simulink model "Filter_testaus_uusi"  (R2017b)
settings: Solver=FixedStepDiscrete  StartTime=0.0  StopTime=10  FixedStep=1/44100  RelTol=1e-3
(part 1 of 4)
settings Model: Creator=Jouni  LastModifiedBy=Jouni
settings CodeAppCC: StateflowObjectComments=on
settings ConfigComp: PLC_TargetIDE=twincat3  PLC_GenerateReport=off  PLC_LaunchReport=off

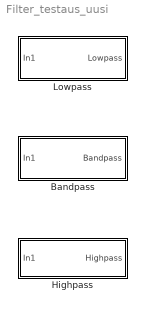
== system Filter_testaus_uusi ==
  Bandpass : Subsystem  TreatAsAtomicUnit=on
  Highpass : Subsystem  TreatAsAtomicUnit=on
  Lowpass : Subsystem  TreatAsAtomicUnit=on

== system Filter_testaus_uusi/Bandpass ==
  In1 : Inport
  BandpassH : Subsystem
  Complex to Real-Imag1 : ComplexToRealImag
  Sum3 : Sum
  Bandpass : Outport
  wires:
  Complex to Real-Imag1/2 -> Sum3/2
  BandpassH/1(Out1) -> Complex to Real-Imag1/1
  Sum3/1 -> Bandpass/1  "Bandpass"
  Complex to Real-Imag1/1 -> Sum3/1
  In1/1 -> BandpassH/1(In1)

== system Filter_testaus_uusi/Highpass ==
  In1 : Inport
  Complex to Real-Imag2 : ComplexToRealImag
  HighpassH : Subsystem
  Sum4 : Sum
  Highpass : Outport
  wires:
  Complex to Real-Imag2/2 -> Sum4/2
  HighpassH/1(Out1) -> Complex to Real-Imag2/1
  Complex to Real-Imag2/1 -> Sum4/1
  Sum4/1 -> Highpass/1  "Highpass"
  In1/1 -> HighpassH/1(In1)

== system Filter_testaus_uusi/Lowpass ==
  In1 : Inport
  Complex to Real-Imag : ComplexToRealImag
  Filter1 : Subsystem  Tag=FilterWizardSubSystem  TreatAsAtomicUnit=on
      settings: ErrorFcn=dspFilterRealizedInBasicElemsAlgLoopErrFcnCallback
  Gain : Gain  Gain=0.75
  LowpassH : Subsystem
  Sum2 : Sum
  Lowpass : Outport
  wires:
  Complex to Real-Imag/2 -> Sum2/2
  LowpassH/1(Out1) -> Complex to Real-Imag/1
  Complex to Real-Imag/1 -> Sum2/1
  Gain/1 -> Filter1/1(Input)
  Sum2/1 -> Lowpass/1  "Lowpass"
  Filter1/1(Output) -> LowpassH/1(In1)
  In1/1 -> Gain/1

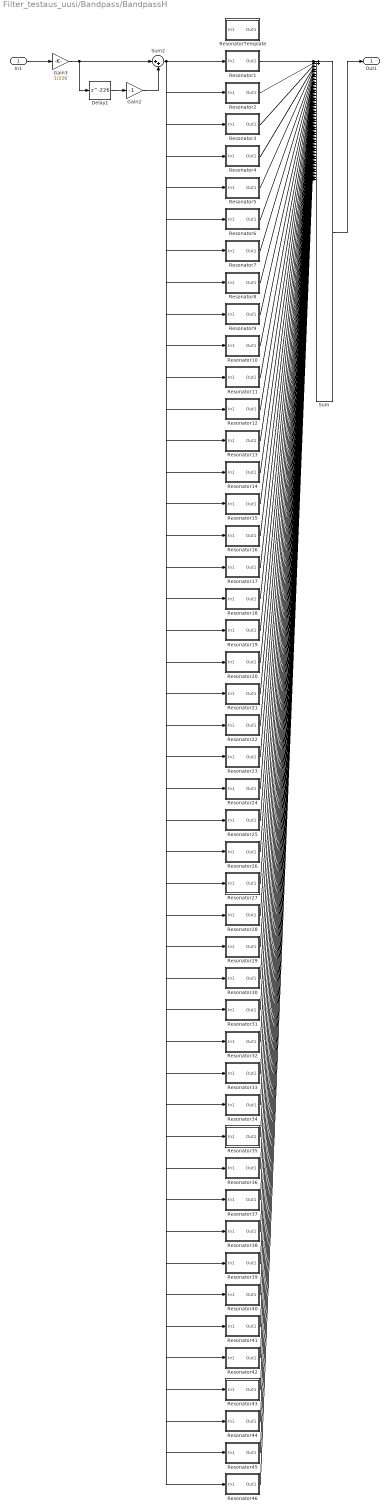
== system Filter_testaus_uusi/Bandpass/BandpassH ==
  In1 : Inport
  Delay1 : Delay  DelayLength=226
  Gain2 : Gain  Gain=-1
  Gain3 : Gain  Gain=1/226
  Resonator1 : Subsystem
  Resonator10 : Subsystem
  Resonator11 : Subsystem
  Resonator12 : Subsystem
  Resonator13 : Subsystem
  Resonator14 : Subsystem
  Resonator15 : Subsystem
  Resonator16 : Subsystem
  Resonator17 : Subsystem
  Resonator18 : Subsystem
  Resonator19 : Subsystem
  Resonator2 : Subsystem
  Resonator20 : Subsystem
  Resonator21 : Subsystem
  Resonator22 : Subsystem
  Resonator23 : Subsystem
  Resonator24 : Subsystem
  Resonator25 : Subsystem
  Resonator26 : Subsystem
  Resonator27 : Subsystem
  Resonator28 : Subsystem
  Resonator29 : Subsystem
  Resonator3 : Subsystem
  Resonator30 : Subsystem
  Resonator31 : Subsystem
  Resonator32 : Subsystem
  Resonator33 : Subsystem
  Resonator34 : Subsystem
  Resonator35 : Subsystem
  Resonator36 : Subsystem
  Resonator37 : Subsystem
  Resonator38 : Subsystem
  Resonator39 : Subsystem
  Resonator4 : Subsystem
  Resonator40 : Subsystem
  Resonator41 : Subsystem
  Resonator42 : Subsystem
  Resonator43 : Subsystem
  Resonator44 : Subsystem
  Resonator45 : Subsystem
  Resonator46 : Subsystem
  Resonator5 : Subsystem
  Resonator6 : Subsystem
  Resonator7 : Subsystem
  Resonator8 : Subsystem
  Resonator9 : Subsystem
  ResonatorTemplate : Subsystem
  Sum : Sum  Inputs=<binary blob, 130 chars, not shown>
  Sum2 : Sum  Inputs=|++
  Out1 : Outport
  wires:
  Delay1/1 -> Gain2/1
  Gain3/1 -> Sum2/1, Delay1/1
  Gain2/1 -> Sum2/2
  In1/1 -> Gain3/1
  Sum/1 -> Out1/1
  Sum2/1 -> Resonator1/1(In1), Resonator2/1(In1), Resonator3/1(In1), Resonator4/1(In1), Resonator5/1(In1), Resonator6/1(In1), Resonator7/1(In1), Resonator8/1(In1), Resonator9/1(In1), Resonator10/1(In1), Resonator11/1(In1), Resonator12/1(In1), Resonator13/1(In1), Resonator14/1(In1), Resonator15/1(In1), Resonator16/1(In1), Resonator17/1(In1), Resonator18/1(In1), Resonator19/1(In1), Resonator20/1(In1), Resonator21/1(In1), Resonator22/1(In1), Resonator23/1(In1), Resonator24/1(In1), Resonator25/1(In1), Resonator26/1(In1), Resonator27/1(In1), Resonator28/1(In1), Resonator29/1(In1), Resonator30/1(In1), Resonator31/1(In1), Resonator32/1(In1), Resonator33/1(In1), Resonator34/1(In1), Resonator35/1(In1), Resonator36/1(In1), Resonator37/1(In1), Resonator38/1(In1), Resonator39/1(In1), Resonator40/1(In1), Resonator41/1(In1), Resonator42/1(In1), Resonator43/1(In1), Resonator44/1(In1), Resonator45/1(In1), Resonator46/1(In1)
  Resonator1/1(Out1) -> Sum/1
  Resonator2/1(Out1) -> Sum/2
  Resonator3/1(Out1) -> Sum/3
  Resonator4/1(Out1) -> Sum/4
  Resonator5/1(Out1) -> Sum/5
  Resonator6/1(Out1) -> Sum/6
  Resonator7/1(Out1) -> Sum/7
  Resonator8/1(Out1) -> Sum/8
  Resonator9/1(Out1) -> Sum/9
  Resonator10/1(Out1) -> Sum/10
  Resonator11/1(Out1) -> Sum/11
  Resonator12/1(Out1) -> Sum/12
  Resonator13/1(Out1) -> Sum/13
  Resonator14/1(Out1) -> Sum/14
  Resonator15/1(Out1) -> Sum/15
  Resonator16/1(Out1) -> Sum/16
  Resonator17/1(Out1) -> Sum/17
  Resonator18/1(Out1) -> Sum/18
  Resonator19/1(Out1) -> Sum/19
  Resonator20/1(Out1) -> Sum/20
  Resonator21/1(Out1) -> Sum/21
  Resonator22/1(Out1) -> Sum/22
  Resonator23/1(Out1) -> Sum/23
  Resonator24/1(Out1) -> Sum/24
  Resonator25/1(Out1) -> Sum/25
  Resonator26/1(Out1) -> Sum/26
  Resonator27/1(Out1) -> Sum/27
  Resonator28/1(Out1) -> Sum/28
  Resonator29/1(Out1) -> Sum/29
  Resonator30/1(Out1) -> Sum/30
  Resonator31/1(Out1) -> Sum/31
  Resonator32/1(Out1) -> Sum/32
  Resonator33/1(Out1) -> Sum/33
  Resonator34/1(Out1) -> Sum/34
  Resonator35/1(Out1) -> Sum/35
  Resonator36/1(Out1) -> Sum/36
  Resonator37/1(Out1) -> Sum/37
  Resonator38/1(Out1) -> Sum/38
  Resonator39/1(Out1) -> Sum/39
  Resonator40/1(Out1) -> Sum/40
  Resonator41/1(Out1) -> Sum/41
  Resonator42/1(Out1) -> Sum/42
  Resonator43/1(Out1) -> Sum/43
  Resonator44/1(Out1) -> Sum/44
  Resonator45/1(Out1) -> Sum/45
  Resonator46/1(Out1) -> Sum/46

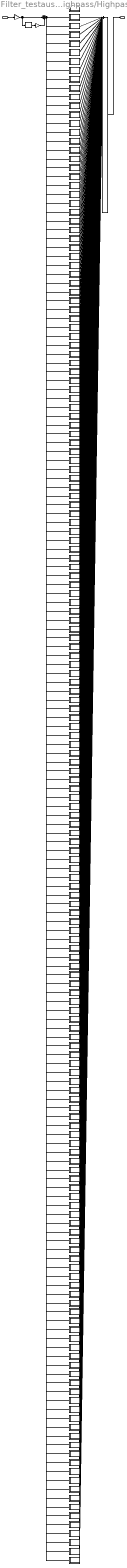
== system Filter_testaus_uusi/Highpass/HighpassH ==
  In1 : Inport
  Delay1 : Delay  DelayLength=226
  Gain2 : Gain  Gain=-1
  Gain3 : Gain  Gain=1/226
  Resonator1 : Subsystem
  Resonator10 : Subsystem
  Resonator100 : Subsystem
  Resonator101 : Subsystem
  Resonator102 : Subsystem
  Resonator103 : Subsystem
  Resonator104 : Subsystem
  Resonator105 : Subsystem
  Resonator106 : Subsystem
  Resonator107 : Subsystem
  Resonator108 : Subsystem
  Resonator109 : Subsystem
  Resonator11 : Subsystem
  Resonator110 : Subsystem
  Resonator111 : Subsystem
  Resonator112 : Subsystem
  Resonator113 : Subsystem
  Resonator114 : Subsystem
  Resonator115 : Subsystem
  Resonator116 : Subsystem
  Resonator117 : Subsystem
  Resonator118 : Subsystem
  Resonator119 : Subsystem
  Resonator12 : Subsystem
  Resonator120 : Subsystem
  Resonator121 : Subsystem
  Resonator122 : Subsystem
  Resonator123 : Subsystem
  Resonator124 : Subsystem
  Resonator125 : Subsystem
  Resonator126 : Subsystem
  Resonator127 : Subsystem
  Resonator128 : Subsystem
  Resonator129 : Subsystem
  Resonator13 : Subsystem
  Resonator130 : Subsystem
  Resonator131 : Subsystem
  Resonator132 : Subsystem
  Resonator133 : Subsystem
  Resonator134 : Subsystem
  Resonator135 : Subsystem
  Resonator136 : Subsystem
  Resonator137 : Subsystem
  Resonator138 : Subsystem
  Resonator139 : Subsystem
  Resonator14 : Subsystem
  Resonator140 : Subsystem
  Resonator141 : Subsystem
  Resonator142 : Subsystem
  Resonator143 : Subsystem
  Resonator144 : Subsystem
  Resonator145 : Subsystem
  Resonator146 : Subsystem
  Resonator147 : Subsystem
  Resonator148 : Subsystem
  Resonator149 : Subsystem
  Resonator15 : Subsystem
  Resonator150 : Subsystem
  Resonator151 : Subsystem
  Resonator152 : Subsystem
  Resonator153 : Subsystem
  Resonator154 : Subsystem
  Resonator155 : Subsystem
  Resonator156 : Subsystem
  Resonator157 : Subsystem
  Resonator158 : Subsystem
  Resonator159 : Subsystem
  Resonator16 : Subsystem
  Resonator160 : Subsystem
  Resonator161 : Subsystem
  Resonator162 : Subsystem
  Resonator163 : Subsystem
  Resonator164 : Subsystem
  Resonator165 : Subsystem
  Resonator166 : Subsystem
  Resonator167 : Subsystem
  Resonator168 : Subsystem
  Resonator169 : Subsystem
  Resonator17 : Subsystem
  Resonator170 : Subsystem
  Resonator171 : Subsystem
  Resonator172 : Subsystem
  Resonator173 : Subsystem
  Resonator174 : Subsystem
  Resonator175 : Subsystem
  Resonator18 : Subsystem
  Resonator19 : Subsystem
  Resonator2 : Subsystem
  Resonator20 : Subsystem
  Resonator21 : Subsystem
  Resonator22 : Subsystem
  Resonator23 : Subsystem
  Resonator24 : Subsystem
  Resonator25 : Subsystem
  Resonator26 : Subsystem
  Resonator27 : Subsystem
  Resonator28 : Subsystem
  Resonator29 : Subsystem
  Resonator3 : Subsystem
  Resonator30 : Subsystem
  Resonator31 : Subsystem
  Resonator32 : Subsystem
  Resonator33 : Subsystem
  Resonator34 : Subsystem
  Resonator35 : Subsystem
  Resonator36 : Subsystem
  Resonator37 : Subsystem
  Resonator38 : Subsystem
  Resonator39 : Subsystem
  Resonator4 : Subsystem
  Resonator40 : Subsystem
  Resonator41 : Subsystem
  Resonator42 : Subsystem
  Resonator43 : Subsystem
  Resonator44 : Subsystem
  Resonator45 : Subsystem
  Resonator46 : Subsystem
  Resonator47 : Subsystem
  Resonator48 : Subsystem
  Resonator49 : Subsystem
  Resonator5 : Subsystem
  Resonator50 : Subsystem
  Resonator51 : Subsystem
  Resonator52 : Subsystem
  Resonator53 : Subsystem
  Resonator54 : Subsystem
  Resonator55 : Subsystem
  Resonator56 : Subsystem
  Resonator57 : Subsystem
  Resonator58 : Subsystem
  Resonator59 : Subsystem
  Resonator6 : Subsystem
  Resonator60 : Subsystem
  Resonator61 : Subsystem
  Resonator62 : Subsystem
  Resonator63 : Subsystem
  Resonator64 : Subsystem
  Resonator65 : Subsystem
  Resonator66 : Subsystem
  Resonator67 : Subsystem
  Resonator68 : Subsystem
  Resonator69 : Subsystem
  Resonator7 : Subsystem
  Resonator70 : Subsystem
  Resonator71 : Subsystem
  Resonator72 : Subsystem
  Resonator73 : Subsystem
  Resonator74 : Subsystem
  Resonator75 : Subsystem
  Resonator76 : Subsystem
  Resonator77 : Subsystem
  Resonator78 : Subsystem
  Resonator79 : Subsystem
  Resonator8 : Subsystem
  Resonator80 : Subsystem
  Resonator81 : Subsystem
  Resonator82 : Subsystem
  Resonator83 : Subsystem
  Resonator84 : Subsystem
  Resonator85 : Subsystem
  Resonator86 : Subsystem
  Resonator87 : Subsystem
  Resonator88 : Subsystem
  Resonator89 : Subsystem
  Resonator9 : Subsystem
  Resonator90 : Subsystem
  Resonator91 : Subsystem
  Resonator92 : Subsystem
  Resonator93 : Subsystem
  Resonator94 : Subsystem
  Resonator95 : Subsystem
  Resonator96 : Subsystem
  Resonator97 : Subsystem
  Resonator98 : Subsystem
  Resonator99 : Subsystem
  ResonatorTemplate : Subsystem
  Sum : Sum  Inputs=<binary blob, 265 chars, not shown>
  Sum2 : Sum  Inputs=|++
  Out1 : Outport
  wires:
  In1/1 -> Gain3/1
  Gain3/1 -> Delay1/1, Sum2/1
  Delay1/1 -> Gain2/1
  Sum/1 -> Out1/1
  Gain2/1 -> Sum2/2
  Sum2/1 -> Resonator1/1(In1), Resonator2/1(In1), Resonator3/1(In1), Resonator4/1(In1), Resonator5/1(In1), Resonator6/1(In1), Resonator7/1(In1), Resonator8/1(In1), Resonator9/1(In1), Resonator10/1(In1), Resonator11/1(In1), Resonator12/1(In1), Resonator13/1(In1), Resonator14/1(In1), Resonator15/1(In1), Resonator16/1(In1), Resonator17/1(In1), Resonator18/1(In1), Resonator19/1(In1), Resonator20/1(In1), Resonator21/1(In1), Resonator22/1(In1), Resonator23/1(In1), Resonator24/1(In1), Resonator25/1(In1), Resonator26/1(In1), Resonator27/1(In1), Resonator28/1(In1), Resonator29/1(In1), Resonator30/1(In1), Resonator31/1(In1), Resonator32/1(In1), Resonator33/1(In1), Resonator34/1(In1), Resonator35/1(In1), Resonator36/1(In1), Resonator37/1(In1), Resonator38/1(In1), Resonator39/1(In1), Resonator40/1(In1), Resonator41/1(In1), Resonator42/1(In1), Resonator43/1(In1), Resonator44/1(In1), Resonator45/1(In1), Resonator46/1(In1), Resonator47/1(In1), Resonator48/1(In1), Resonator49/1(In1), Resonator50/1(In1), Resonator51/1(In1), Resonator52/1(In1), Resonator53/1(In1), Resonator54/1(In1), Resonator55/1(In1), Resonator56/1(In1), Resonator57/1(In1), Resonator58/1(In1), Resonator59/1(In1), Resonator60/1(In1), Resonator61/1(In1), Resonator62/1(In1), Resonator63/1(In1), Resonator64/1(In1), Resonator65/1(In1), Resonator66/1(In1), Resonator67/1(In1), Resonator68/1(In1), Resonator69/1(In1), Resonator70/1(In1), Resonator71/1(In1), Resonator72/1(In1), Resonator73/1(In1), Resonator74/1(In1), Resonator75/1(In1), Resonator76/1(In1), Resonator77/1(In1), Resonator78/1(In1), Resonator79/1(In1), Resonator80/1(In1), Resonator81/1(In1), Resonator82/1(In1), Resonator83/1(In1), Resonator84/1(In1), Resonator85/1(In1), Resonator86/1(In1), Resonator87/1(In1), Resonator88/1(In1), Resonator89/1(In1), Resonator90/1(In1), Resonator91/1(In1), Resonator92/1(In1), Resonator93/1(In1), Resonator94/1(In1), Resonator95/1(In1), Resonator96/1(In1), Resonator97/1(In1), Resonator98/1(In1), Resonator99/1(In1), Resonator100/1(In1), Resonator101/1(In1), Resonator102/1(In1), Resonator103/1(In1), Resonator104/1(In1), Resonator105/1(In1), Resonator106/1(In1), Resonator107/1(In1), Resonator108/1(In1), Resonator109/1(In1), Resonator110/1(In1), Resonator111/1(In1), Resonator112/1(In1), Resonator113/1(In1), Resonator114/1(In1), Resonator115/1(In1), Resonator116/1(In1), Resonator117/1(In1), Resonator118/1(In1), Resonator119/1(In1), Resonator120/1(In1), Resonator121/1(In1), Resonator122/1(In1), Resonator123/1(In1), Resonator124/1(In1), Resonator125/1(In1), Resonator126/1(In1), Resonator127/1(In1), Resonator128/1(In1), Resonator129/1(In1), Resonator130/1(In1), Resonator131/1(In1), Resonator132/1(In1), Resonator133/1(In1), Resonator134/1(In1), Resonator135/1(In1), Resonator136/1(In1), Resonator137/1(In1), Resonator138/1(In1), Resonator139/1(In1), Resonator140/1(In1), Resonator141/1(In1), Resonator142/1(In1), Resonator143/1(In1), Resonator144/1(In1), Resonator145/1(In1), Resonator146/1(In1), Resonator147/1(In1), Resonator148/1(In1), Resonator149/1(In1), Resonator150/1(In1), Resonator151/1(In1), Resonator152/1(In1), Resonator153/1(In1), Resonator154/1(In1), Resonator155/1(In1), Resonator156/1(In1), Resonator157/1(In1), Resonator158/1(In1), Resonator159/1(In1), Resonator160/1(In1), Resonator161/1(In1), Resonator162/1(In1), Resonator163/1(In1), Resonator164/1(In1), Resonator165/1(In1), Resonator166/1(In1), Resonator167/1(In1), Resonator168/1(In1), Resonator169/1(In1), Resonator170/1(In1), Resonator171/1(In1), Resonator172/1(In1), Resonator173/1(In1), Resonator174/1(In1), Resonator175/1(In1)
  Resonator1/1(Out1) -> Sum/1
  Resonator2/1(Out1) -> Sum/2
  Resonator3/1(Out1) -> Sum/3
  Resonator4/1(Out1) -> Sum/4
  Resonator5/1(Out1) -> Sum/5
  Resonator6/1(Out1) -> Sum/6
  Resonator7/1(Out1) -> Sum/7
  Resonator8/1(Out1) -> Sum/8
  Resonator9/1(Out1) -> Sum/9
  Resonator10/1(Out1) -> Sum/10
  Resonator11/1(Out1) -> Sum/11
  Resonator12/1(Out1) -> Sum/12
  Resonator13/1(Out1) -> Sum/13
  Resonator14/1(Out1) -> Sum/14
  Resonator15/1(Out1) -> Sum/15
  Resonator16/1(Out1) -> Sum/16
  Resonator17/1(Out1) -> Sum/17
  Resonator18/1(Out1) -> Sum/18
  Resonator19/1(Out1) -> Sum/19
  Resonator20/1(Out1) -> Sum/20
  Resonator21/1(Out1) -> Sum/21
  Resonator22/1(Out1) -> Sum/22
  Resonator23/1(Out1) -> Sum/23
  Resonator24/1(Out1) -> Sum/24
  Resonator25/1(Out1) -> Sum/25
  Resonator26/1(Out1) -> Sum/26
  Resonator27/1(Out1) -> Sum/27
  Resonator28/1(Out1) -> Sum/28
  Resonator29/1(Out1) -> Sum/29
  Resonator30/1(Out1) -> Sum/30
  Resonator31/1(Out1) -> Sum/31
  Resonator32/1(Out1) -> Sum/32
  Resonator33/1(Out1) -> Sum/33
  Resonator34/1(Out1) -> Sum/34
  Resonator35/1(Out1) -> Sum/35
  Resonator36/1(Out1) -> Sum/36
  Resonator37/1(Out1) -> Sum/37
  Resonator38/1(Out1) -> Sum/38
  Resonator39/1(Out1) -> Sum/39
  Resonator40/1(Out1) -> Sum/40
  Resonator41/1(Out1) -> Sum/41
  Resonator42/1(Out1) -> Sum/42
  Resonator43/1(Out1) -> Sum/43
  Resonator44/1(Out1) -> Sum/44
  Resonator45/1(Out1) -> Sum/45
  Resonator46/1(Out1) -> Sum/46
  Resonator47/1(Out1) -> Sum/47
  Resonator48/1(Out1) -> Sum/48
  Resonator49/1(Out1) -> Sum/49
  Resonator50/1(Out1) -> Sum/50
  Resonator51/1(Out1) -> Sum/51
  Resonator52/1(Out1) -> Sum/52
  Resonator53/1(Out1) -> Sum/53
  Resonator54/1(Out1) -> Sum/54
  Resonator55/1(Out1) -> Sum/55
  Resonator56/1(Out1) -> Sum/56
  Resonator57/1(Out1) -> Sum/57
  Resonator58/1(Out1) -> Sum/58
  Resonator59/1(Out1) -> Sum/59
  Resonator60/1(Out1) -> Sum/60
  Resonator61/1(Out1) -> Sum/61
  Resonator62/1(Out1) -> Sum/62
  Resonator63/1(Out1) -> Sum/63
  Resonator64/1(Out1) -> Sum/64
  Resonator65/1(Out1) -> Sum/65
  Resonator66/1(Out1) -> Sum/66
  Resonator67/1(Out1) -> Sum/67
  Resonator68/1(Out1) -> Sum/68
  Resonator69/1(Out1) -> Sum/69
  Resonator70/1(Out1) -> Sum/70
  Resonator71/1(Out1) -> Sum/71
  Resonator72/1(Out1) -> Sum/72
  Resonator73/1(Out1) -> Sum/73
  Resonator74/1(Out1) -> Sum/74
  Resonator75/1(Out1) -> Sum/75
  Resonator76/1(Out1) -> Sum/76
  Resonator77/1(Out1) -> Sum/77
  Resonator78/1(Out1) -> Sum/78
  Resonator79/1(Out1) -> Sum/79
  Resonator80/1(Out1) -> Sum/80
  Resonator81/1(Out1) -> Sum/81
  Resonator82/1(Out1) -> Sum/82
  Resonator83/1(Out1) -> Sum/83
  Resonator84/1(Out1) -> Sum/84
  Resonator85/1(Out1) -> Sum/85
  Resonator86/1(Out1) -> Sum/86
  Resonator87/1(Out1) -> Sum/87
  Resonator88/1(Out1) -> Sum/88
  Resonator89/1(Out1) -> Sum/89
  Resonator90/1(Out1) -> Sum/90
  Resonator91/1(Out1) -> Sum/91
  Resonator92/1(Out1) -> Sum/92
  Resonator93/1(Out1) -> Sum/93
  Resonator94/1(Out1) -> Sum/94
  Resonator95/1(Out1) -> Sum/95
  Resonator96/1(Out1) -> Sum/96
  Resonator97/1(Out1) -> Sum/97
  Resonator98/1(Out1) -> Sum/98
  Resonator99/1(Out1) -> Sum/99
  Resonator100/1(Out1) -> Sum/100
  Resonator101/1(Out1) -> Sum/101
  Resonator102/1(Out1) -> Sum/102
  Resonator103/1(Out1) -> Sum/103
  Resonator104/1(Out1) -> Sum/104
  Resonator105/1(Out1) -> Sum/105
  Resonator106/1(Out1) -> Sum/106
  Resonator107/1(Out1) -> Sum/107
  Resonator108/1(Out1) -> Sum/108
  Resonator109/1(Out1) -> Sum/109
  Resonator110/1(Out1) -> Sum/110
  Resonator111/1(Out1) -> Sum/111
  Resonator112/1(Out1) -> Sum/112
  Resonator113/1(Out1) -> Sum/113
  Resonator114/1(Out1) -> Sum/114
  Resonator115/1(Out1) -> Sum/115
  Resonator116/1(Out1) -> Sum/116
  Resonator117/1(Out1) -> Sum/117
  Resonator118/1(Out1) -> Sum/118
  Resonator119/1(Out1) -> Sum/119
  Resonator120/1(Out1) -> Sum/120
  Resonator121/1(Out1) -> Sum/121
  Resonator122/1(Out1) -> Sum/122
  Resonator123/1(Out1) -> Sum/123
  Resonator124/1(Out1) -> Sum/124
  Resonator125/1(Out1) -> Sum/125
  Resonator126/1(Out1) -> Sum/126
  Resonator127/1(Out1) -> Sum/127
  Resonator128/1(Out1) -> Sum/128
  Resonator129/1(Out1) -> Sum/129
  Resonator130/1(Out1) -> Sum/130
  Resonator131/1(Out1) -> Sum/131
  Resonator132/1(Out1) -> Sum/132
  Resonator133/1(Out1) -> Sum/133
  Resonator134/1(Out1) -> Sum/134
  Resonator135/1(Out1) -> Sum/135
  Resonator136/1(Out1) -> Sum/136
  Resonator137/1(Out1) -> Sum/137
  Resonator138/1(Out1) -> Sum/138
  Resonator139/1(Out1) -> Sum/139
  Resonator140/1(Out1) -> Sum/140
  Resonator141/1(Out1) -> Sum/141
  Resonator142/1(Out1) -> Sum/142
  Resonator143/1(Out1) -> Sum/143
  Resonator144/1(Out1) -> Sum/144
  Resonator145/1(Out1) -> Sum/145
  Resonator146/1(Out1) -> Sum/146
  Resonator147/1(Out1) -> Sum/147
  Resonator148/1(Out1) -> Sum/148
  Resonator149/1(Out1) -> Sum/149
  Resonator150/1(Out1) -> Sum/150
  Resonator151/1(Out1) -> Sum/151
  Resonator152/1(Out1) -> Sum/152
  Resonator153/1(Out1) -> Sum/153
  Resonator154/1(Out1) -> Sum/154
  Resonator155/1(Out1) -> Sum/155
  Resonator156/1(Out1) -> Sum/156
  Resonator157/1(Out1) -> Sum/157
  Resonator158/1(Out1) -> Sum/158
  Resonator159/1(Out1) -> Sum/159
  Resonator160/1(Out1) -> Sum/160
  Resonator161/1(Out1) -> Sum/161
  Resonator162/1(Out1) -> Sum/162
  Resonator163/1(Out1) -> Sum/163
  Resonator164/1(Out1) -> Sum/164
  Resonator165/1(Out1) -> Sum/165
  Resonator166/1(Out1) -> Sum/166
  Resonator167/1(Out1) -> Sum/167
  Resonator168/1(Out1) -> Sum/168
  Resonator169/1(Out1) -> Sum/169
  Resonator170/1(Out1) -> Sum/170
  Resonator171/1(Out1) -> Sum/171
  Resonator172/1(Out1) -> Sum/172
  Resonator173/1(Out1) -> Sum/173
  Resonator174/1(Out1) -> Sum/174
  Resonator175/1(Out1) -> Sum/175

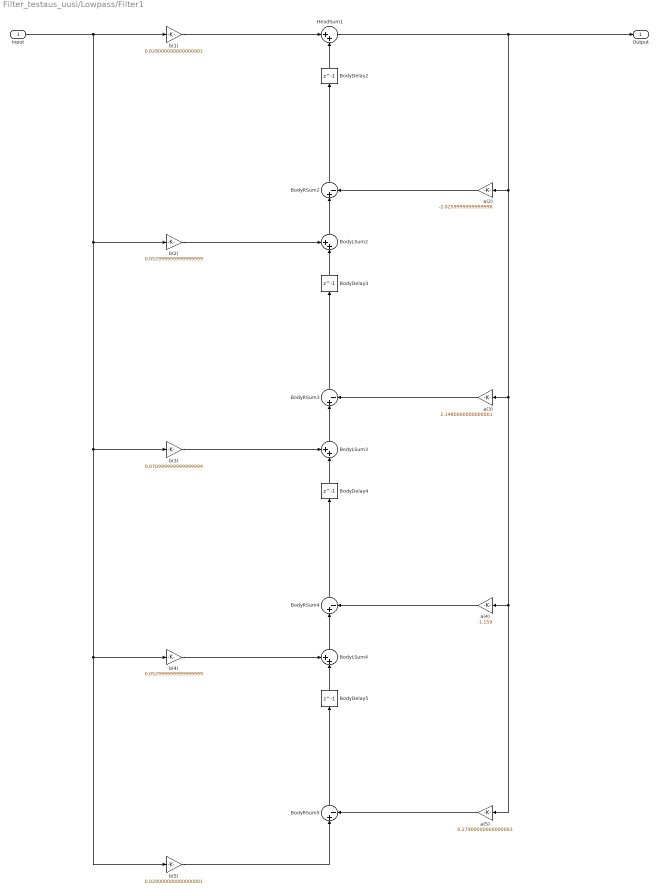
== system Filter_testaus_uusi/Lowpass/Filter1 ==
  Input : Inport
  BodyDelay{2..5} (4 alike) : Delay  DelayLength=1  InitialCondition=0
  BodyLSum2 : Sum  Inputs=++|  RndMeth=Nearest  SaturateOnIntegerOverflow=on  OutDataTypeStr=Inherit: Same as first input
  BodyLSum3 : Sum  Inputs=++|  RndMeth=Nearest  SaturateOnIntegerOverflow=on  OutDataTypeStr=Inherit: Same as first input
  BodyLSum4 : Sum  Inputs=++|  RndMeth=Nearest  SaturateOnIntegerOverflow=on  OutDataTypeStr=Inherit: Same as first input
  BodyRSum{2..5} (4 alike) : Sum  Inputs=|+-  RndMeth=Nearest  SaturateOnIntegerOverflow=on  OutDataTypeStr=Inherit: Same as first input
  HeadSum1 : Sum  Inputs=|++  RndMeth=Nearest  SaturateOnIntegerOverflow=on  OutDataTypeStr=Inherit: Same as first input
  a(2) : Gain  Gain=-2.0259999999999998  ParamDataTypeStr=double  RndMeth=Nearest  SaturateOnIntegerOverflow=on  OutDataTypeStr=Inherit: Same as input
  a(3) : Gain  Gain=2.1480000000000001  ParamDataTypeStr=double  RndMeth=Nearest  SaturateOnIntegerOverflow=on  OutDataTypeStr=Inherit: Same as input
  a(4) : Gain  Gain=-1.159  ParamDataTypeStr=double  RndMeth=Nearest  SaturateOnIntegerOverflow=on  OutDataTypeStr=Inherit: Same as input
  a(5) : Gain  Gain=0.27900000000000003  ParamDataTypeStr=double  RndMeth=Nearest  SaturateOnIntegerOverflow=on  OutDataTypeStr=Inherit: Same as input
  b(1) : Gain  Gain=0.028000000000000001  ParamDataTypeStr=double  RndMeth=Nearest  SaturateOnIntegerOverflow=on  OutDataTypeStr=Inherit: Same as input
  b(2) : Gain  Gain=0.052999999999999999  ParamDataTypeStr=double  RndMeth=Nearest  SaturateOnIntegerOverflow=on  OutDataTypeStr=Inherit: Same as input
  b(3) : Gain  Gain=0.070999999999999994  ParamDataTypeStr=double  RndMeth=Nearest  SaturateOnIntegerOverflow=on  OutDataTypeStr=Inherit: Same as input
  b(4) : Gain  Gain=0.052999999999999999  ParamDataTypeStr=double  RndMeth=Nearest  SaturateOnIntegerOverflow=on  OutDataTypeStr=Inherit: Same as input
  b(5) : Gain  Gain=0.028000000000000001  ParamDataTypeStr=double  RndMeth=Nearest  SaturateOnIntegerOverflow=on  OutDataTypeStr=Inherit: Same as input
  Output : Outport
  wires:
  Input/1 -> b(4)/1, b(5)/1, b(3)/1, b(2)/1, b(1)/1
  b(1)/1 -> HeadSum1/1
  HeadSum1/1 -> a(4)/1, a(5)/1, a(3)/1, a(2)/1, Output/1
  b(2)/1 -> BodyLSum2/1
  BodyLSum2/1 -> BodyRSum2/1
  BodyRSum2/1 -> BodyDelay2/1
  a(2)/1 -> BodyRSum2/2
  BodyDelay2/1 -> HeadSum1/2
  b(3)/1 -> BodyLSum3/1
  BodyLSum3/1 -> BodyRSum3/1
  BodyRSum3/1 -> BodyDelay3/1
  a(3)/1 -> BodyRSum3/2
  BodyDelay3/1 -> BodyLSum2/2
  b(4)/1 -> BodyLSum4/1
  BodyLSum4/1 -> BodyRSum4/1
  BodyRSum4/1 -> BodyDelay4/1
  a(4)/1 -> BodyRSum4/2
  BodyDelay4/1 -> BodyLSum3/2
  b(5)/1 -> BodyRSum5/1
  BodyRSum5/1 -> BodyDelay5/1
  a(5)/1 -> BodyRSum5/2
  BodyDelay5/1 -> BodyLSum4/2

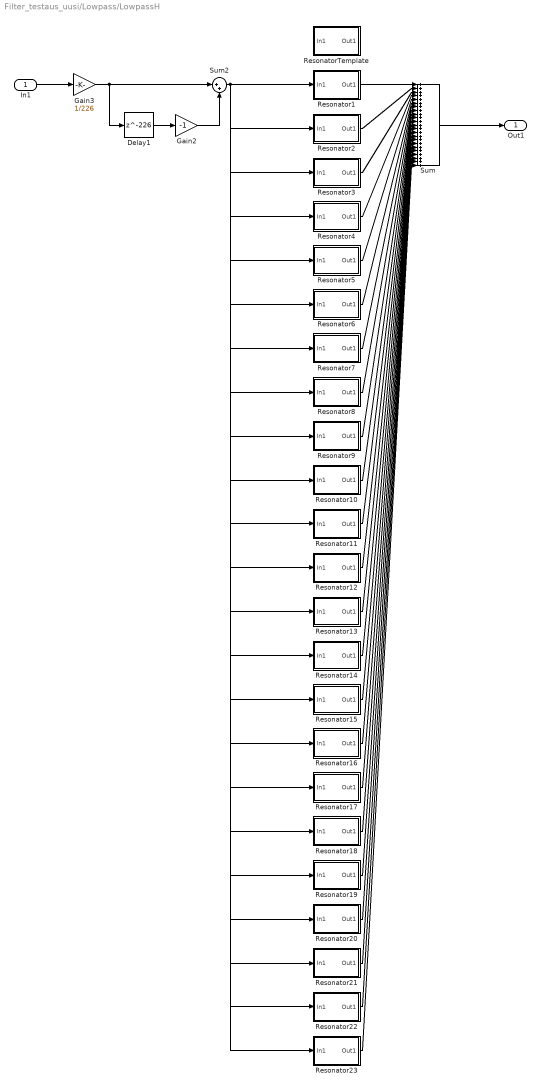
== system Filter_testaus_uusi/Lowpass/LowpassH ==
  In1 : Inport
  Delay1 : Delay  DelayLength=226
  Gain2 : Gain  Gain=-1
  Gain3 : Gain  Gain=1/226
  Resonator1 : Subsystem
  Resonator10 : Subsystem
  Resonator11 : Subsystem
  Resonator12 : Subsystem
  Resonator13 : Subsystem
  Resonator14 : Subsystem
  Resonator15 : Subsystem
  Resonator16 : Subsystem
  Resonator17 : Subsystem
  Resonator18 : Subsystem
  Resonator19 : Subsystem
  Resonator2 : Subsystem
  Resonator20 : Subsystem
  Resonator21 : Subsystem
  Resonator22 : Subsystem
  Resonator23 : Subsystem
  Resonator3 : Subsystem
  Resonator4 : Subsystem
  Resonator5 : Subsystem
  Resonator6 : Subsystem
  Resonator7 : Subsystem
  Resonator8 : Subsystem
  Resonator9 : Subsystem
  ResonatorTemplate : Subsystem
  Sum : Sum  Inputs=+++++++++++++++++++++++
  Sum2 : Sum  Inputs=|++
  Out1 : Outport
  wires:
  In1/1 -> Gain3/1
  Gain2/1 -> Sum2/2
  Gain3/1 -> Delay1/1, Sum2/1
  Delay1/1 -> Gain2/1
  Sum/1 -> Out1/1
  Sum2/1 -> Resonator1/1(In1), Resonator2/1(In1), Resonator3/1(In1), Resonator4/1(In1), Resonator5/1(In1), Resonator6/1(In1), Resonator7/1(In1), Resonator8/1(In1), Resonator9/1(In1), Resonator10/1(In1), Resonator11/1(In1), Resonator12/1(In1), Resonator13/1(In1), Resonator14/1(In1), Resonator15/1(In1), Resonator16/1(In1), Resonator17/1(In1), Resonator18/1(In1), Resonator19/1(In1), Resonator20/1(In1), Resonator21/1(In1), Resonator22/1(In1), Resonator23/1(In1)
  Resonator1/1(Out1) -> Sum/1
  Resonator2/1(Out1) -> Sum/2
  Resonator3/1(Out1) -> Sum/3
  Resonator4/1(Out1) -> Sum/4
  Resonator5/1(Out1) -> Sum/5
  Resonator6/1(Out1) -> Sum/6
  Resonator7/1(Out1) -> Sum/7
  Resonator8/1(Out1) -> Sum/8
  Resonator9/1(Out1) -> Sum/9
  Resonator10/1(Out1) -> Sum/10
  Resonator11/1(Out1) -> Sum/11
  Resonator12/1(Out1) -> Sum/12
  Resonator13/1(Out1) -> Sum/13
  Resonator14/1(Out1) -> Sum/14
  Resonator15/1(Out1) -> Sum/15
  Resonator16/1(Out1) -> Sum/16
  Resonator17/1(Out1) -> Sum/17
  Resonator18/1(Out1) -> Sum/18
  Resonator19/1(Out1) -> Sum/19
  Resonator20/1(Out1) -> Sum/20
  Resonator21/1(Out1) -> Sum/21
  Resonator22/1(Out1) -> Sum/22
  Resonator23/1(Out1) -> Sum/23

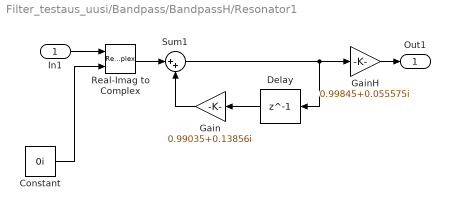
== system Filter_testaus_uusi/Bandpass/BandpassH/Resonator1 ==
  In1 : Inport
  Constant : Constant  Value=0i
  Delay : Delay  DelayLength=1
  Gain : Gain  Gain=0.99035+0.13856i
  GainH : Gain  Gain=0.99845+0.055575i
  Real-Imag to Complex : RealImagToComplex
  Sum1 : Sum  Inputs=|++
  Out1 : Outport
  wires:
  Constant/1 -> Real-Imag to Complex/2
  Real-Imag to Complex/1 -> Sum1/1
  In1/1 -> Real-Imag to Complex/1
  GainH/1 -> Out1/1
  Gain/1 -> Sum1/2
  Delay/1 -> Gain/1
  Sum1/1 -> Delay/1, GainH/1

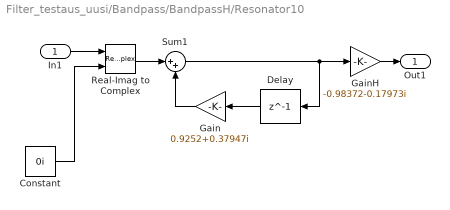
== system Filter_testaus_uusi/Bandpass/BandpassH/Resonator10 ==
  In1 : Inport
  Constant : Constant  Value=0i
  Delay : Delay  DelayLength=1
  Gain : Gain  Gain=0.9252+0.37947i
  GainH : Gain  Gain=-0.98372-0.17973i
  Real-Imag to Complex : RealImagToComplex
  Sum1 : Sum  Inputs=|++
  Out1 : Outport
  wires:
  Constant/1 -> Real-Imag to Complex/2
  Real-Imag to Complex/1 -> Sum1/1
  In1/1 -> Real-Imag to Complex/1
  GainH/1 -> Out1/1
  Gain/1 -> Sum1/2
  Delay/1 -> Gain/1
  Sum1/1 -> Delay/1, GainH/1

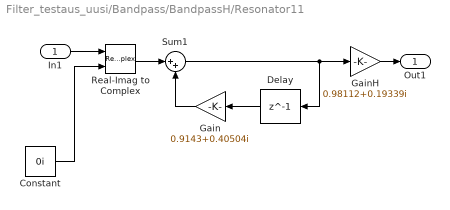
== system Filter_testaus_uusi/Bandpass/BandpassH/Resonator11 ==
  In1 : Inport
  Constant : Constant  Value=0i
  Delay : Delay  DelayLength=1
  Gain : Gain  Gain=0.9143+0.40504i
  GainH : Gain  Gain=0.98112+0.19339i
  Real-Imag to Complex : RealImagToComplex
  Sum1 : Sum  Inputs=|++
  Out1 : Outport
  wires:
  Constant/1 -> Real-Imag to Complex/2
  Real-Imag to Complex/1 -> Sum1/1
  In1/1 -> Real-Imag to Complex/1
  GainH/1 -> Out1/1
  Gain/1 -> Sum1/2
  Delay/1 -> Gain/1
  Sum1/1 -> Delay/1, GainH/1

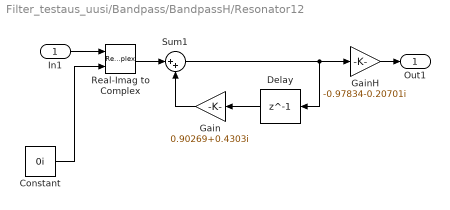
== system Filter_testaus_uusi/Bandpass/BandpassH/Resonator12 ==
  In1 : Inport
  Constant : Constant  Value=0i
  Delay : Delay  DelayLength=1
  Gain : Gain  Gain=0.90269+0.4303i
  GainH : Gain  Gain=-0.97834-0.20701i
  Real-Imag to Complex : RealImagToComplex
  Sum1 : Sum  Inputs=|++
  Out1 : Outport
  wires:
  Constant/1 -> Real-Imag to Complex/2
  Real-Imag to Complex/1 -> Sum1/1
  In1/1 -> Real-Imag to Complex/1
  GainH/1 -> Out1/1
  Gain/1 -> Sum1/2
  Delay/1 -> Gain/1
  Sum1/1 -> Delay/1, GainH/1

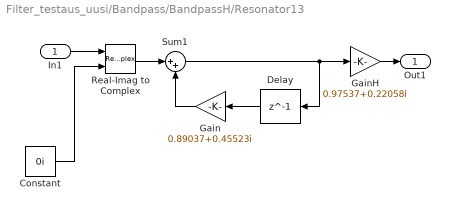
== system Filter_testaus_uusi/Bandpass/BandpassH/Resonator13 ==
  In1 : Inport
  Constant : Constant  Value=0i
  Delay : Delay  DelayLength=1
  Gain : Gain  Gain=0.89037+0.45523i
  GainH : Gain  Gain=0.97537+0.22058i
  Real-Imag to Complex : RealImagToComplex
  Sum1 : Sum  Inputs=|++
  Out1 : Outport
  wires:
  Constant/1 -> Real-Imag to Complex/2
  Real-Imag to Complex/1 -> Sum1/1
  In1/1 -> Real-Imag to Complex/1
  GainH/1 -> Out1/1
  Gain/1 -> Sum1/2
  Delay/1 -> Gain/1
  Sum1/1 -> Delay/1, GainH/1

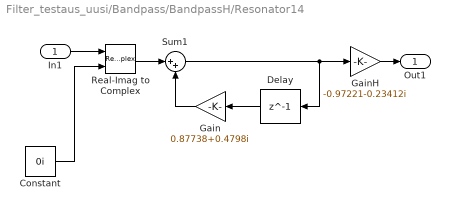
== system Filter_testaus_uusi/Bandpass/BandpassH/Resonator14 ==
  In1 : Inport
  Constant : Constant  Value=0i
  Delay : Delay  DelayLength=1
  Gain : Gain  Gain=0.87738+0.4798i
  GainH : Gain  Gain=-0.97221-0.23412i
  Real-Imag to Complex : RealImagToComplex
  Sum1 : Sum  Inputs=|++
  Out1 : Outport
  wires:
  Constant/1 -> Real-Imag to Complex/2
  Real-Imag to Complex/1 -> Sum1/1
  In1/1 -> Real-Imag to Complex/1
  GainH/1 -> Out1/1
  Gain/1 -> Sum1/2
  Delay/1 -> Gain/1
  Sum1/1 -> Delay/1, GainH/1

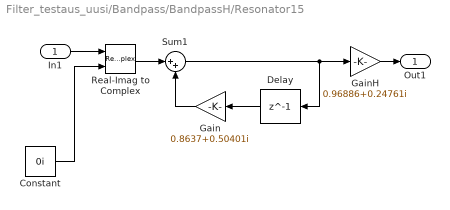
== system Filter_testaus_uusi/Bandpass/BandpassH/Resonator15 ==
  In1 : Inport
  Constant : Constant  Value=0i
  Delay : Delay  DelayLength=1
  Gain : Gain  Gain=0.8637+0.50401i
  GainH : Gain  Gain=0.96886+0.24761i
  Real-Imag to Complex : RealImagToComplex
  Sum1 : Sum  Inputs=|++
  Out1 : Outport
  wires:
  Constant/1 -> Real-Imag to Complex/2
  Real-Imag to Complex/1 -> Sum1/1
  In1/1 -> Real-Imag to Complex/1
  GainH/1 -> Out1/1
  Gain/1 -> Sum1/2
  Delay/1 -> Gain/1
  Sum1/1 -> Delay/1, GainH/1

== system Filter_testaus_uusi/Bandpass/BandpassH/Resonator16 ==
  In1 : Inport
  Constant : Constant  Value=0i
  Delay : Delay  DelayLength=1
  Gain : Gain  Gain=0.84936+0.52782i
  GainH : Gain  Gain=-0.96532-0.26106i
  Real-Imag to Complex : RealImagToComplex
  Sum1 : Sum  Inputs=|++
  Out1 : Outport
  wires:
  Constant/1 -> Real-Imag to Complex/2
  Real-Imag to Complex/1 -> Sum1/1
  In1/1 -> Real-Imag to Complex/1
  GainH/1 -> Out1/1
  Gain/1 -> Sum1/2
  Delay/1 -> Gain/1
  Sum1/1 -> Delay/1, GainH/1

== system Filter_testaus_uusi/Bandpass/BandpassH/Resonator17 ==
  In1 : Inport
  Constant : Constant  Value=0i
  Delay : Delay  DelayLength=1
  Gain : Gain  Gain=0.83435+0.55123i
  GainH : Gain  Gain=0.9616+0.27445i
  Real-Imag to Complex : RealImagToComplex
  Sum1 : Sum  Inputs=|++
  Out1 : Outport
  wires:
  Constant/1 -> Real-Imag to Complex/2
  Real-Imag to Complex/1 -> Sum1/1
  In1/1 -> Real-Imag to Complex/1
  GainH/1 -> Out1/1
  Gain/1 -> Sum1/2
  Delay/1 -> Gain/1
  Sum1/1 -> Delay/1, GainH/1

== system Filter_testaus_uusi/Bandpass/BandpassH/Resonator18 ==
  In1 : Inport
  Constant : Constant  Value=0i
  Delay : Delay  DelayLength=1
  Gain : Gain  Gain=0.81871+0.57421i
  GainH : Gain  Gain=-0.95769-0.28779i
  Real-Imag to Complex : RealImagToComplex
  Sum1 : Sum  Inputs=|++
  Out1 : Outport
  wires:
  Constant/1 -> Real-Imag to Complex/2
  Real-Imag to Complex/1 -> Sum1/1
  In1/1 -> Real-Imag to Complex/1
  GainH/1 -> Out1/1
  Gain/1 -> Sum1/2
  Delay/1 -> Gain/1
  Sum1/1 -> Delay/1, GainH/1

== system Filter_testaus_uusi/Bandpass/BandpassH/Resonator19 ==
  In1 : Inport
  Constant : Constant  Value=0i
  Delay : Delay  DelayLength=1
  Gain : Gain  Gain=0.80243+0.59675i
  GainH : Gain  Gain=0.9536+0.30107i
  Real-Imag to Complex : RealImagToComplex
  Sum1 : Sum  Inputs=|++
  Out1 : Outport
  wires:
  Constant/1 -> Real-Imag to Complex/2
  Real-Imag to Complex/1 -> Sum1/1
  In1/1 -> Real-Imag to Complex/1
  GainH/1 -> Out1/1
  Gain/1 -> Sum1/2
  Delay/1 -> Gain/1
  Sum1/1 -> Delay/1, GainH/1

== system Filter_testaus_uusi/Bandpass/BandpassH/Resonator2 ==
  In1 : Inport
  Constant : Constant  Value=0i
  Delay : Delay  DelayLength=1
  Gain : Gain  Gain=0.98612+0.16604i
  GainH : Gain  Gain=-0.99759-0.069448i
  Real-Imag to Complex : RealImagToComplex
  Sum1 : Sum  Inputs=|++
  Out1 : Outport
  wires:
  Constant/1 -> Real-Imag to Complex/2
  Real-Imag to Complex/1 -> Sum1/1
  In1/1 -> Real-Imag to Complex/1
  GainH/1 -> Out1/1
  Gain/1 -> Sum1/2
  Delay/1 -> Gain/1
  Sum1/1 -> Delay/1, GainH/1

== system Filter_testaus_uusi/Bandpass/BandpassH/Resonator20 ==
  In1 : Inport
  Constant : Constant  Value=0i
  Delay : Delay  DelayLength=1
  Gain : Gain  Gain=0.78553+0.61882i
  GainH : Gain  Gain=-0.94932-0.3143i
  Real-Imag to Complex : RealImagToComplex
  Sum1 : Sum  Inputs=|++
  Out1 : Outport
  wires:
  Constant/1 -> Real-Imag to Complex/2
  Real-Imag to Complex/1 -> Sum1/1
  In1/1 -> Real-Imag to Complex/1
  GainH/1 -> Out1/1
  Gain/1 -> Sum1/2
  Delay/1 -> Gain/1
  Sum1/1 -> Delay/1, GainH/1

== system Filter_testaus_uusi/Bandpass/BandpassH/Resonator21 ==
  In1 : Inport
  Constant : Constant  Value=0i
  Delay : Delay  DelayLength=1
  Gain : Gain  Gain=0.76803+0.64042i
  GainH : Gain  Gain=0.94486+0.32747i
  Real-Imag to Complex : RealImagToComplex
  Sum1 : Sum  Inputs=|++
  Out1 : Outport
  wires:
  Constant/1 -> Real-Imag to Complex/2
  Real-Imag to Complex/1 -> Sum1/1
  In1/1 -> Real-Imag to Complex/1
  GainH/1 -> Out1/1
  Gain/1 -> Sum1/2
  Delay/1 -> Gain/1
  Sum1/1 -> Delay/1, GainH/1

== system Filter_testaus_uusi/Bandpass/BandpassH/Resonator22 ==
  In1 : Inport
  Constant : Constant  Value=0i
  Delay : Delay  DelayLength=1
  Gain : Gain  Gain=0.74993+0.66152i
  GainH : Gain  Gain=-0.94022-0.34057i
  Real-Imag to Complex : RealImagToComplex
  Sum1 : Sum  Inputs=|++
  Out1 : Outport
  wires:
  Constant/1 -> Real-Imag to Complex/2
  Real-Imag to Complex/1 -> Sum1/1
  In1/1 -> Real-Imag to Complex/1
  GainH/1 -> Out1/1
  Gain/1 -> Sum1/2
  Delay/1 -> Gain/1
  Sum1/1 -> Delay/1, GainH/1

== system Filter_testaus_uusi/Bandpass/BandpassH/Resonator23 ==
  In1 : Inport
  Constant : Constant  Value=0i
  Delay : Delay  DelayLength=1
  Gain : Gain  Gain=0.73125+0.68211i
  GainH : Gain  Gain=0.93539+0.3536i
  Real-Imag to Complex : RealImagToComplex
  Sum1 : Sum  Inputs=|++
  Out1 : Outport
  wires:
  Constant/1 -> Real-Imag to Complex/2
  Real-Imag to Complex/1 -> Sum1/1
  In1/1 -> Real-Imag to Complex/1
  GainH/1 -> Out1/1
  Gain/1 -> Sum1/2
  Delay/1 -> Gain/1
  Sum1/1 -> Delay/1, GainH/1

== system Filter_testaus_uusi/Bandpass/BandpassH/Resonator24 ==
  In1 : Inport
  Constant : Constant  Value=0i
  Delay : Delay  DelayLength=1
  Gain : Gain  Gain=0.76803-0.64042i
  GainH : Gain  Gain=0.93539-0.3536i
  Real-Imag to Complex : RealImagToComplex
  Sum1 : Sum  Inputs=|++
  Out1 : Outport
  wires:
  Constant/1 -> Real-Imag to Complex/2
  Real-Imag to Complex/1 -> Sum1/1
  In1/1 -> Real-Imag to Complex/1
  GainH/1 -> Out1/1
  Gain/1 -> Sum1/2
  Delay/1 -> Gain/1
  Sum1/1 -> Delay/1, GainH/1

== system Filter_testaus_uusi/Bandpass/BandpassH/Resonator25 ==
  In1 : Inport
  Constant : Constant  Value=0i
  Delay : Delay  DelayLength=1
  Gain : Gain  Gain=0.78553-0.61882i
  GainH : Gain  Gain=-0.94022+0.34057i
  Real-Imag to Complex : RealImagToComplex
  Sum1 : Sum  Inputs=|++
  Out1 : Outport
  wires:
  Constant/1 -> Real-Imag to Complex/2
  Real-Imag to Complex/1 -> Sum1/1
  In1/1 -> Real-Imag to Complex/1
  GainH/1 -> Out1/1
  Gain/1 -> Sum1/2
  Delay/1 -> Gain/1
  Sum1/1 -> Delay/1, GainH/1

== system Filter_testaus_uusi/Bandpass/BandpassH/Resonator26 ==
  In1 : Inport
  Constant : Constant  Value=0i
  Delay : Delay  DelayLength=1
  Gain : Gain  Gain=0.80243-0.59675i
  GainH : Gain  Gain=0.94486-0.32747i
  Real-Imag to Complex : RealImagToComplex
  Sum1 : Sum  Inputs=|++
  Out1 : Outport
  wires:
  Constant/1 -> Real-Imag to Complex/2
  Real-Imag to Complex/1 -> Sum1/1
  In1/1 -> Real-Imag to Complex/1
  GainH/1 -> Out1/1
  Gain/1 -> Sum1/2
  Delay/1 -> Gain/1
  Sum1/1 -> Delay/1, GainH/1

== system Filter_testaus_uusi/Bandpass/BandpassH/Resonator27 ==
  In1 : Inport
  Constant : Constant  Value=0i
  Delay : Delay  DelayLength=1
  Gain : Gain  Gain=0.81871-0.57421i
  GainH : Gain  Gain=-0.94932+0.3143i
  Real-Imag to Complex : RealImagToComplex
  Sum1 : Sum  Inputs=|++
  Out1 : Outport
  wires:
  Constant/1 -> Real-Imag to Complex/2
  Real-Imag to Complex/1 -> Sum1/1
  In1/1 -> Real-Imag to Complex/1
  GainH/1 -> Out1/1
  Gain/1 -> Sum1/2
  Delay/1 -> Gain/1
  Sum1/1 -> Delay/1, GainH/1

== system Filter_testaus_uusi/Bandpass/BandpassH/Resonator28 ==
  In1 : Inport
  Constant : Constant  Value=0i
  Delay : Delay  DelayLength=1
  Gain : Gain  Gain=0.83435-0.55123i
  GainH : Gain  Gain=0.9536-0.30107i
  Real-Imag to Complex : RealImagToComplex
  Sum1 : Sum  Inputs=|++
  Out1 : Outport
  wires:
  Constant/1 -> Real-Imag to Complex/2
  Real-Imag to Complex/1 -> Sum1/1
  In1/1 -> Real-Imag to Complex/1
  GainH/1 -> Out1/1
  Gain/1 -> Sum1/2
  Delay/1 -> Gain/1
  Sum1/1 -> Delay/1, GainH/1

== system Filter_testaus_uusi/Bandpass/BandpassH/Resonator29 ==
  In1 : Inport
  Constant : Constant  Value=0i
  Delay : Delay  DelayLength=1
  Gain : Gain  Gain=0.84936-0.52782i
  GainH : Gain  Gain=-0.95769+0.28779i
  Real-Imag to Complex : RealImagToComplex
  Sum1 : Sum  Inputs=|++
  Out1 : Outport
  wires:
  Constant/1 -> Real-Imag to Complex/2
  Real-Imag to Complex/1 -> Sum1/1
  In1/1 -> Real-Imag to Complex/1
  GainH/1 -> Out1/1
  Gain/1 -> Sum1/2
  Delay/1 -> Gain/1
  Sum1/1 -> Delay/1, GainH/1

== system Filter_testaus_uusi/Bandpass/BandpassH/Resonator3 ==
  In1 : Inport
  Constant : Constant  Value=0i
  Delay : Delay  DelayLength=1
  Gain : Gain  Gain=0.98112+0.19339i
  GainH : Gain  Gain=0.99652+0.083308i
  Real-Imag to Complex : RealImagToComplex
  Sum1 : Sum  Inputs=|++
  Out1 : Outport
  wires:
  Constant/1 -> Real-Imag to Complex/2
  Real-Imag to Complex/1 -> Sum1/1
  In1/1 -> Real-Imag to Complex/1
  GainH/1 -> Out1/1
  Gain/1 -> Sum1/2
  Delay/1 -> Gain/1
  Sum1/1 -> Delay/1, GainH/1

== system Filter_testaus_uusi/Bandpass/BandpassH/Resonator30 ==
  In1 : Inport
  Constant : Constant  Value=0i
  Delay : Delay  DelayLength=1
  Gain : Gain  Gain=0.8637-0.50401i
  GainH : Gain  Gain=0.9616-0.27445i
  Real-Imag to Complex : RealImagToComplex
  Sum1 : Sum  Inputs=|++
  Out1 : Outport
  wires:
  Constant/1 -> Real-Imag to Complex/2
  Real-Imag to Complex/1 -> Sum1/1
  In1/1 -> Real-Imag to Complex/1
  GainH/1 -> Out1/1
  Gain/1 -> Sum1/2
  Delay/1 -> Gain/1
  Sum1/1 -> Delay/1, GainH/1

== system Filter_testaus_uusi/Bandpass/BandpassH/Resonator31 ==
  In1 : Inport
  Constant : Constant  Value=0i
  Delay : Delay  DelayLength=1
  Gain : Gain  Gain=0.87738-0.4798i
  GainH : Gain  Gain=-0.96532+0.26106i
  Real-Imag to Complex : RealImagToComplex
  Sum1 : Sum  Inputs=|++
  Out1 : Outport
  wires:
  Constant/1 -> Real-Imag to Complex/2
  Real-Imag to Complex/1 -> Sum1/1
  In1/1 -> Real-Imag to Complex/1
  GainH/1 -> Out1/1
  Gain/1 -> Sum1/2
  Delay/1 -> Gain/1
  Sum1/1 -> Delay/1, GainH/1

== system Filter_testaus_uusi/Bandpass/BandpassH/Resonator32 ==
  In1 : Inport
  Constant : Constant  Value=0i
  Delay : Delay  DelayLength=1
  Gain : Gain  Gain=0.89037-0.45523i
  GainH : Gain  Gain=0.96886-0.24761i
  Real-Imag to Complex : RealImagToComplex
  Sum1 : Sum  Inputs=|++
  Out1 : Outport
  wires:
  Constant/1 -> Real-Imag to Complex/2
  Real-Imag to Complex/1 -> Sum1/1
  In1/1 -> Real-Imag to Complex/1
  GainH/1 -> Out1/1
  Gain/1 -> Sum1/2
  Delay/1 -> Gain/1
  Sum1/1 -> Delay/1, GainH/1

== system Filter_testaus_uusi/Bandpass/BandpassH/Resonator33 ==
  In1 : Inport
  Constant : Constant  Value=0i
  Delay : Delay  DelayLength=1
  Gain : Gain  Gain=0.90269-0.4303i
  GainH : Gain  Gain=-0.97221+0.23412i
  Real-Imag to Complex : RealImagToComplex
  Sum1 : Sum  Inputs=|++
  Out1 : Outport
  wires:
  Constant/1 -> Real-Imag to Complex/2
  Real-Imag to Complex/1 -> Sum1/1
  In1/1 -> Real-Imag to Complex/1
  GainH/1 -> Out1/1
  Gain/1 -> Sum1/2
  Delay/1 -> Gain/1
  Sum1/1 -> Delay/1, GainH/1

== system Filter_testaus_uusi/Bandpass/BandpassH/Resonator34 ==
  In1 : Inport
  Constant : Constant  Value=0i
  Delay : Delay  DelayLength=1
  Gain : Gain  Gain=0.9143-0.40504i
  GainH : Gain  Gain=0.97537-0.22058i
  Real-Imag to Complex : RealImagToComplex
  Sum1 : Sum  Inputs=|++
  Out1 : Outport
  wires:
  Constant/1 -> Real-Imag to Complex/2
  Real-Imag to Complex/1 -> Sum1/1
  In1/1 -> Real-Imag to Complex/1
  GainH/1 -> Out1/1
  Gain/1 -> Sum1/2
  Delay/1 -> Gain/1
  Sum1/1 -> Delay/1, GainH/1

== system Filter_testaus_uusi/Bandpass/BandpassH/Resonator35 ==
  In1 : Inport
  Constant : Constant  Value=0i
  Delay : Delay  DelayLength=1
  Gain : Gain  Gain=0.9252-0.37947i
  GainH : Gain  Gain=-0.97834+0.20701i
  Real-Imag to Complex : RealImagToComplex
  Sum1 : Sum  Inputs=|++
  Out1 : Outport
  wires:
  Constant/1 -> Real-Imag to Complex/2
  Real-Imag to Complex/1 -> Sum1/1
  In1/1 -> Real-Imag to Complex/1
  GainH/1 -> Out1/1
  Gain/1 -> Sum1/2
  Delay/1 -> Gain/1
  Sum1/1 -> Delay/1, GainH/1

== system Filter_testaus_uusi/Bandpass/BandpassH/Resonator36 ==
  In1 : Inport
  Constant : Constant  Value=0i
  Delay : Delay  DelayLength=1
  Gain : Gain  Gain=0.93539-0.3536i
  GainH : Gain  Gain=0.98112-0.19339i
  Real-Imag to Complex : RealImagToComplex
  Sum1 : Sum  Inputs=|++
  Out1 : Outport
  wires:
  Constant/1 -> Real-Imag to Complex/2
  Real-Imag to Complex/1 -> Sum1/1
  In1/1 -> Real-Imag to Complex/1
  GainH/1 -> Out1/1
  Gain/1 -> Sum1/2
  Delay/1 -> Gain/1
  Sum1/1 -> Delay/1, GainH/1

== system Filter_testaus_uusi/Bandpass/BandpassH/Resonator37 ==
  In1 : Inport
  Constant : Constant  Value=0i
  Delay : Delay  DelayLength=1
  Gain : Gain  Gain=0.94486-0.32747i
  GainH : Gain  Gain=-0.98372+0.17973i
  Real-Imag to Complex : RealImagToComplex
  Sum1 : Sum  Inputs=|++
  Out1 : Outport
  wires:
  Constant/1 -> Real-Imag to Complex/2
  Real-Imag to Complex/1 -> Sum1/1
  In1/1 -> Real-Imag to Complex/1
  GainH/1 -> Out1/1
  Gain/1 -> Sum1/2
  Delay/1 -> Gain/1
  Sum1/1 -> Delay/1, GainH/1

== system Filter_testaus_uusi/Bandpass/BandpassH/Resonator38 ==
  In1 : Inport
  Constant : Constant  Value=0i
  Delay : Delay  DelayLength=1
  Gain : Gain  Gain=0.9536-0.30107i
  GainH : Gain  Gain=0.98612-0.16604i
  Real-Imag to Complex : RealImagToComplex
  Sum1 : Sum  Inputs=|++
  Out1 : Outport
  wires:
  Constant/1 -> Real-Imag to Complex/2
  Real-Imag to Complex/1 -> Sum1/1
  In1/1 -> Real-Imag to Complex/1
  GainH/1 -> Out1/1
  Gain/1 -> Sum1/2
  Delay/1 -> Gain/1
  Sum1/1 -> Delay/1, GainH/1

== system Filter_testaus_uusi/Bandpass/BandpassH/Resonator39 ==
  In1 : Inport
  Constant : Constant  Value=0i
  Delay : Delay  DelayLength=1
  Gain : Gain  Gain=0.9616-0.27445i
  GainH : Gain  Gain=-0.98833+0.15231i
  Real-Imag to Complex : RealImagToComplex
  Sum1 : Sum  Inputs=|++
  Out1 : Outport
  wires:
  Constant/1 -> Real-Imag to Complex/2
  Real-Imag to Complex/1 -> Sum1/1
  In1/1 -> Real-Imag to Complex/1
  GainH/1 -> Out1/1
  Gain/1 -> Sum1/2
  Delay/1 -> Gain/1
  Sum1/1 -> Delay/1, GainH/1

== system Filter_testaus_uusi/Bandpass/BandpassH/Resonator4 ==
  In1 : Inport
  Constant : Constant  Value=0i
  Delay : Delay  DelayLength=1
  Gain : Gain  Gain=0.97537+0.22058i
  GainH : Gain  Gain=-0.99527-0.097152i
  Real-Imag to Complex : RealImagToComplex
  Sum1 : Sum  Inputs=|++
  Out1 : Outport
  wires:
  Constant/1 -> Real-Imag to Complex/2
  Real-Imag to Complex/1 -> Sum1/1
  In1/1 -> Real-Imag to Complex/1
  GainH/1 -> Out1/1
  Gain/1 -> Sum1/2
  Delay/1 -> Gain/1
  Sum1/1 -> Delay/1, GainH/1

== system Filter_testaus_uusi/Bandpass/BandpassH/Resonator40 ==
  In1 : Inport
  Constant : Constant  Value=0i
  Delay : Delay  DelayLength=1
  Gain : Gain  Gain=0.96886-0.24761i
  GainH : Gain  Gain=0.99035-0.13856i
  Real-Imag to Complex : RealImagToComplex
  Sum1 : Sum  Inputs=|++
  Out1 : Outport
  wires:
  Constant/1 -> Real-Imag to Complex/2
  Real-Imag to Complex/1 -> Sum1/1
  In1/1 -> Real-Imag to Complex/1
  GainH/1 -> Out1/1
  Gain/1 -> Sum1/2
  Delay/1 -> Gain/1
  Sum1/1 -> Delay/1, GainH/1

== system Filter_testaus_uusi/Bandpass/BandpassH/Resonator41 ==
  In1 : Inport
  Constant : Constant  Value=0i
  Delay : Delay  DelayLength=1
  Gain : Gain  Gain=0.97537-0.22058i
  GainH : Gain  Gain=-0.99218+0.12478i
  Real-Imag to Complex : RealImagToComplex
  Sum1 : Sum  Inputs=|++
  Out1 : Outport
  wires:
  Constant/1 -> Real-Imag to Complex/2
  Real-Imag to Complex/1 -> Sum1/1
  In1/1 -> Real-Imag to Complex/1
  GainH/1 -> Out1/1
  Gain/1 -> Sum1/2
  Delay/1 -> Gain/1
  Sum1/1 -> Delay/1, GainH/1

== system Filter_testaus_uusi/Bandpass/BandpassH/Resonator42 ==
  In1 : Inport
  Constant : Constant  Value=0i
  Delay : Delay  DelayLength=1
  Gain : Gain  Gain=0.98112-0.19339i
  GainH : Gain  Gain=0.99382-0.11098i
  Real-Imag to Complex : RealImagToComplex
  Sum1 : Sum  Inputs=|++
  Out1 : Outport
  wires:
  Constant/1 -> Real-Imag to Complex/2
  Real-Imag to Complex/1 -> Sum1/1
  In1/1 -> Real-Imag to Complex/1
  GainH/1 -> Out1/1
  Gain/1 -> Sum1/2
  Delay/1 -> Gain/1
  Sum1/1 -> Delay/1, GainH/1

== system Filter_testaus_uusi/Bandpass/BandpassH/Resonator43 ==
  In1 : Inport
  Constant : Constant  Value=0i
  Delay : Delay  DelayLength=1
  Gain : Gain  Gain=0.98612-0.16604i
  GainH : Gain  Gain=-0.99527+0.097152i
  Real-Imag to Complex : RealImagToComplex
  Sum1 : Sum  Inputs=|++
  Out1 : Outport
  wires:
  Constant/1 -> Real-Imag to Complex/2
  Real-Imag to Complex/1 -> Sum1/1
  In1/1 -> Real-Imag to Complex/1
  GainH/1 -> Out1/1
  Gain/1 -> Sum1/2
  Delay/1 -> Gain/1
  Sum1/1 -> Delay/1, GainH/1

== system Filter_testaus_uusi/Bandpass/BandpassH/Resonator44 ==
  In1 : Inport
  Constant : Constant  Value=0i
  Delay : Delay  DelayLength=1
  Gain : Gain  Gain=0.99035-0.13856i
  GainH : Gain  Gain=0.99652-0.083308i
  Real-Imag to Complex : RealImagToComplex
  Sum1 : Sum  Inputs=|++
  Out1 : Outport
  wires:
  Constant/1 -> Real-Imag to Complex/2
  Real-Imag to Complex/1 -> Sum1/1
  In1/1 -> Real-Imag to Complex/1
  GainH/1 -> Out1/1
  Gain/1 -> Sum1/2
  Delay/1 -> Gain/1
  Sum1/1 -> Delay/1, GainH/1

== system Filter_testaus_uusi/Bandpass/BandpassH/Resonator45 ==
  In1 : Inport
  Constant : Constant  Value=0i
  Delay : Delay  DelayLength=1
  Gain : Gain  Gain=0.99382-0.11098i
  GainH : Gain  Gain=-0.99759+0.069448i
  Real-Imag to Complex : RealImagToComplex
  Sum1 : Sum  Inputs=|++
  Out1 : Outport
  wires:
  Constant/1 -> Real-Imag to Complex/2
  Real-Imag to Complex/1 -> Sum1/1
  In1/1 -> Real-Imag to Complex/1
  GainH/1 -> Out1/1
  Gain/1 -> Sum1/2
  Delay/1 -> Gain/1
  Sum1/1 -> Delay/1, GainH/1

== system Filter_testaus_uusi/Bandpass/BandpassH/Resonator46 ==
  In1 : Inport
  Constant : Constant  Value=0i
  Delay : Delay  DelayLength=1
  Gain : Gain  Gain=0.99652-0.083308i
  GainH : Gain  Gain=0.99845-0.055575i
  Real-Imag to Complex : RealImagToComplex
  Sum1 : Sum  Inputs=|++
  Out1 : Outport
  wires:
  Constant/1 -> Real-Imag to Complex/2
  Real-Imag to Complex/1 -> Sum1/1
  In1/1 -> Real-Imag to Complex/1
  GainH/1 -> Out1/1
  Gain/1 -> Sum1/2
  Delay/1 -> Gain/1
  Sum1/1 -> Delay/1, GainH/1

== system Filter_testaus_uusi/Bandpass/BandpassH/Resonator5 ==
  In1 : Inport
  Constant : Constant  Value=0i
  Delay : Delay  DelayLength=1
  Gain : Gain  Gain=0.96886+0.24761i
  GainH : Gain  Gain=0.99382+0.11098i
  Real-Imag to Complex : RealImagToComplex
  Sum1 : Sum  Inputs=|++
  Out1 : Outport
  wires:
  Constant/1 -> Real-Imag to Complex/2
  Real-Imag to Complex/1 -> Sum1/1
  In1/1 -> Real-Imag to Complex/1
  GainH/1 -> Out1/1
  Gain/1 -> Sum1/2
  Delay/1 -> Gain/1
  Sum1/1 -> Delay/1, GainH/1

== system Filter_testaus_uusi/Bandpass/BandpassH/Resonator6 ==
  In1 : Inport
  Constant : Constant  Value=0i
  Delay : Delay  DelayLength=1
  Gain : Gain  Gain=0.9616+0.27445i
  GainH : Gain  Gain=-0.99218-0.12478i
  Real-Imag to Complex : RealImagToComplex
  Sum1 : Sum  Inputs=|++
  Out1 : Outport
  wires:
  Constant/1 -> Real-Imag to Complex/2
  Real-Imag to Complex/1 -> Sum1/1
  In1/1 -> Real-Imag to Complex/1
  GainH/1 -> Out1/1
  Gain/1 -> Sum1/2
  Delay/1 -> Gain/1
  Sum1/1 -> Delay/1, GainH/1

== system Filter_testaus_uusi/Bandpass/BandpassH/Resonator7 ==
  In1 : Inport
  Constant : Constant  Value=0i
  Delay : Delay  DelayLength=1
  Gain : Gain  Gain=0.9536+0.30107i
  GainH : Gain  Gain=0.99035+0.13856i
  Real-Imag to Complex : RealImagToComplex
  Sum1 : Sum  Inputs=|++
  Out1 : Outport
  wires:
  Constant/1 -> Real-Imag to Complex/2
  Real-Imag to Complex/1 -> Sum1/1
  In1/1 -> Real-Imag to Complex/1
  GainH/1 -> Out1/1
  Gain/1 -> Sum1/2
  Delay/1 -> Gain/1
  Sum1/1 -> Delay/1, GainH/1

== system Filter_testaus_uusi/Bandpass/BandpassH/Resonator8 ==
  In1 : Inport
  Constant : Constant  Value=0i
  Delay : Delay  DelayLength=1
  Gain : Gain  Gain=0.94486+0.32747i
  GainH : Gain  Gain=-0.98833-0.15231i
  Real-Imag to Complex : RealImagToComplex
  Sum1 : Sum  Inputs=|++
  Out1 : Outport
  wires:
  Constant/1 -> Real-Imag to Complex/2
  Real-Imag to Complex/1 -> Sum1/1
  In1/1 -> Real-Imag to Complex/1
  GainH/1 -> Out1/1
  Gain/1 -> Sum1/2
  Delay/1 -> Gain/1
  Sum1/1 -> Delay/1, GainH/1

== system Filter_testaus_uusi/Bandpass/BandpassH/Resonator9 ==
  In1 : Inport
  Constant : Constant  Value=0i
  Delay : Delay  DelayLength=1
  Gain : Gain  Gain=0.93539+0.3536i
  GainH : Gain  Gain=0.98612+0.16604i
  Real-Imag to Complex : RealImagToComplex
  Sum1 : Sum  Inputs=|++
  Out1 : Outport
  wires:
  Constant/1 -> Real-Imag to Complex/2
  Real-Imag to Complex/1 -> Sum1/1
  In1/1 -> Real-Imag to Complex/1
  GainH/1 -> Out1/1
  Gain/1 -> Sum1/2
  Delay/1 -> Gain/1
  Sum1/1 -> Delay/1, GainH/1

== system Filter_testaus_uusi/Bandpass/BandpassH/ResonatorTemplate ==
  In1 : Inport
  Constant : Constant  Value=0i
  Delay : Delay  DelayLength=1
  Gain : Gain
  GainH : Gain
  Real-Imag to Complex : RealImagToComplex
  Sum1 : Sum  Inputs=|++
  Out1 : Outport
  wires:
  Sum1/1 -> GainH/1, Delay/1
  Delay/1 -> Gain/1
  Gain/1 -> Sum1/2
  GainH/1 -> Out1/1
  In1/1 -> Real-Imag to Complex/1
  Real-Imag to Complex/1 -> Sum1/1
  Constant/1 -> Real-Imag to Complex/2

== system Filter_testaus_uusi/Highpass/HighpassH/Resonator1 ==
  In1 : Inport
  Constant : Constant  Value=0i
  Delay : Delay  DelayLength=1
  Gain : Gain  Gain=0.73125+0.68211i
  GainH : Gain  Gain=0.93539+0.3536i
  Real-Imag to Complex : RealImagToComplex
  Sum1 : Sum  Inputs=|++
  Out1 : Outport
  wires:
  Constant/1 -> Real-Imag to Complex/2
  Real-Imag to Complex/1 -> Sum1/1
  In1/1 -> Real-Imag to Complex/1
  GainH/1 -> Out1/1
  Gain/1 -> Sum1/2
  Delay/1 -> Gain/1
  Sum1/1 -> Delay/1, GainH/1

== system Filter_testaus_uusi/Highpass/HighpassH/Resonator10 ==
  In1 : Inport
  Constant : Constant  Value=0i
  Delay : Delay  DelayLength=1
  Gain : Gain  Gain=0.53958+0.84194i
  GainH : Gain  Gain=-0.88396-0.46756i
  Real-Imag to Complex : RealImagToComplex
  Sum1 : Sum  Inputs=|++
  Out1 : Outport
  wires:
  Constant/1 -> Real-Imag to Complex/2
  Real-Imag to Complex/1 -> Sum1/1
  In1/1 -> Real-Imag to Complex/1
  GainH/1 -> Out1/1
  Gain/1 -> Sum1/2
  Delay/1 -> Gain/1
  Sum1/1 -> Delay/1, GainH/1
